simulink model "pmdc_motor"  (R2022b)
settings: Solver=ode23t  StartTime=0.0  StopTime=0.1  MaxStep=1e-5  RelTol=1e-5  AbsTol=1e-5
values from neighbouring files (symbols this model uses):
  Beq = Bn + Bload    (= 0)    [motor_parameter.m]
  Jeq = Jn + Jload    (= 0.00252)    [motor_parameter.m]
  K = 0.764    [motor_parameter.m]
  La = 3e-3    (= 0.003)    [motor_parameter.m]
  Ra = 0.8    [motor_parameter.m]
  Va_rated = 120    [motor_parameter.m]
libraries: spsControlledVoltageSourceLib x1, spsDCMachineLib x1, cstblocks x1, spspowerguiLib x1
settings Model: Creator=NT550XDA-KC35W  LastModifiedBy=NT550XDA-KC35W

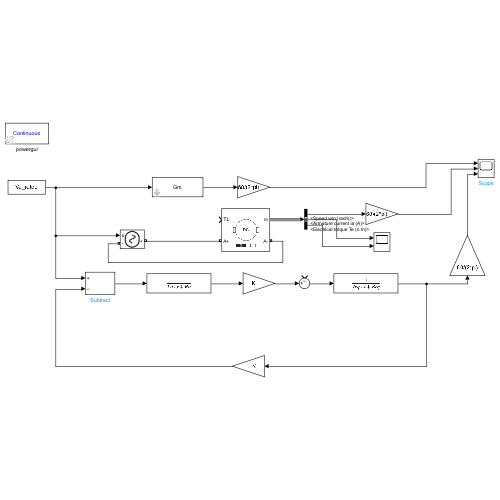
[thumbnail: Simulink's stored preview of the top-level diagram]
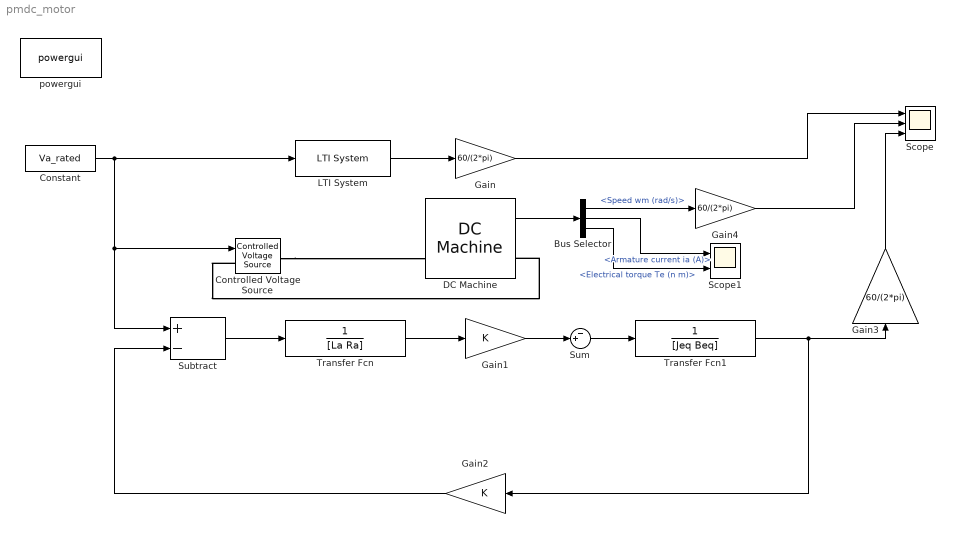
== system pmdc_motor ==
  Bus Selector : BusSelector  OutputSignals=Speed wm (rad/s),Armature current ia (A),Electrical torque Te (n m)
  Constant : Constant  Value=Va_rated
  Controlled Voltage Source : spsControlledVoltageSourceLib/Controlled Voltage Source  Initialize=on  Source_Type=AC  Amplitude=0  Phase=0  Frequency=0  Measurements=None
  DC Machine : spsDCMachineLib/DC Machine  PresetModel=No  MechanicalLoad=Torque TL  FieldType=Permanent magnet  ShowDetailedParameters=on  MeasurementBus=off  RLa="[ Ra  La]"  RLf="[ 240  120]"  Laf=1.8  MachineConstant=Back-emf constant (V/rpm)  Ke=K*2*pi/60  Kt=1.8  J=Jeq  Bm=Beq  Tf=0  w0=0  Ifinit=1  TsPowergui=0  TsBlock=-1
  Gain : Gain  Gain=60/(2*pi)
  Gain1 : Gain  Gain=K
  Gain2 : Gain  Gain=K
  Gain3 : Gain  Gain=60/(2*pi)
  Gain4 : Gain  Gain=60/(2*pi)
  LTI System : cstblocks/LTI System  sys=Gm  IC=[]
  Scope : Scope  NumInputPorts=3
  Scope1 : Scope  NumInputPorts=2
  Subtract : Sum  Inputs=+-
  Sum : Sum  Inputs=-+|
  Transfer Fcn : TransferFcn  Denominator=[La Ra]
  Transfer Fcn1 : TransferFcn  Denominator=[Jeq Beq]
  powergui : spspowerguiLib/powergui  Priority=1  SimulationMode=Continuous  SampleTime=50e-6  frequency=60  Iterations=50  frequencyindice=0  Pbase=100e6  ErrMax=1e-4  UnitsV=kV  UnitsW=MW  buscounter=0  FunctionMessages=off  echomessages=off  EnableUseOfTLC=off  CurrentSourceSwitches=off  DisableSnubberDevices=off  DisableRonSwitches=off  DisableVfSwitches=off  DisplayEquations=off  AutomaticDiscreteSolvers=off  SolverType=Tustin/Backward Euler (TBE)  Interpol=off  ExternalGateDelay=off  methode=off  Ts=100  x0status=blocks  SPID=on  SwTol=0  HookPort=off  NonlinearTolerance=1e-4  nMaxIteration=100  ContinueOnMaxIteration=off  RestoreLinks=warning  ResistiveCurrentMeasurement=off  Frange=[0:2:500]  Ylog=off  Xlog=on  ShowGrid=off  save=off  variable=ZData  structure=0  ZoomFFT=off  StartTime=0.0  cycles=1  DisplayStyle=1  fundamental=60  FreqAxis=off  MaxFrequency=1000  frequencyindicesteady=1  RmsSteady=1  display=off
  wires:
  Constant/1 -> Controlled Voltage Source/1, Subtract/1, LTI System/1
  LTI System/1 -> Gain/1
  Gain/1 -> Scope/1
  Subtract/1 -> Transfer Fcn/1
  Transfer Fcn/1 -> Gain1/1
  Gain1/1 -> Sum/2
  Sum/1 -> Transfer Fcn1/1
  Gain2/1 -> Subtract/2
  Transfer Fcn1/1 -> Gain3/1, Gain2/1
  DC Machine/1 -> Bus Selector/1
  Bus Selector/1 -> Gain4/1  "<Speed wm (rad/s)>"
  Gain4/1 -> Scope/2
  Gain3/1 -> Scope/3
  Bus Selector/2 -> Scope1/1  "<Armature current ia (A)>"
  Bus Selector/3 -> Scope1/2  "<Electrical torque Te (n m)>"
  connections:
  Controlled Voltage Source/RConn1 -- DC Machine/LConn1
  Controlled Voltage Source/LConn1 -- DC Machine/RConn1
